simulink model "AR4FullPositionControl"  (R2026a)
settings: Solver=FixedStepAuto  StopTime=inf  FixedStep=3e-5
PreLoadFcn:
  | load('last_pos.mat');
StopFcn:
  | save('last_pos.mat', 'posJ6', 'posJ5', 'posJ4', 'posJ3', 'posJ2', 'posJ1', 'lastX', 'lastY', 'lastZ');
undefined symbols (not defined in the file): targetColor, targetGo, targetX, targetY, targetZ
libraries: arduinolib x31
(part 2 of 3)

== matlab function AR4FullPositionControl/Subsystem/J6/MATLAB Function1 ==
  data: startNext input; clk input; count output; dt input; rst input; displaySpeed output; dir output; pul output; next output; speedRPM input; positionAngle input; currCount input; accelRPMperSec input; limit output; mode input; homed output
function [count, displaySpeed, dir, pul, next, limit, homed] = J6(startNext, clk, dt, rst, speedRPM, positionAngle, currCount, accelRPMperSec, mode)
% J6 - Joint 6 position/speed controller with S-curve acceleration + HOMING
%
% AR4-MK3 robot. Continuous-rotation wrist joint (+/-180 = same physical spot).
% positionAngle is remapped +180 internally. Switch is at count 0.
%
% MODE:
%   0 = POSITION, 1 = INITIALIZE (drive to HOME_TARGET), 2 = HOMING
%
%   >>> maxCount = 20000   GEAR_RATIO = 20000/4000 = 5.0
%   >>> J6 may sit AT the switch (180/-180); limit only flags on TRUE overtravel.

    persistent currentCount lastClkState lastCount spTimer smoothedSpeed ...
               currentRPM distTraveled totalMoveFrozen lastTarget pulseAccum ...
               homedFlag lastMode;

    % -------------------------------------------------------------------------
    % CONSTANTS
    % -------------------------------------------------------------------------
    Ts           = 3e-5;
    PPR          = 1000;
    CPR          = PPR * 4;
    GEAR_RATIO   = 20000 / CPR;
    maxCount     = 20000;
    LIMIT_BUFFER = 5;        % used for homing/fault logic (NOT target clamp)
    TARGET_MARGIN = 0;       % <<< target clamp margin: 0 = allow reaching both ends
    OVERTRAVEL   = 30;       % <<< counts beyond range before a REAL fault trips
    TUNE_C2R     = 0.8;
    C2R          = (GEAR_RATIO * CPR) / 60 * TUNE_C2R;

    speedUpdateInterval = 0.2;
    ALPHA               = 0.3;
    MIN_RPM             = 0.5;
    STOP_COUNTS         = 1;

    HOME_RPM    = 5;    % <<< tune: slow safe homing speed (RPM)
    HOME_TARGET = 0;    % <<< angle commanded in mode=1, for THIS joint (deg)

    % -------------------------------------------------------------------------
    % INITIALISATION (first call only)
    % -------------------------------------------------------------------------
    if isempty(currentCount)
        currentCount    = currCount;
        lastCount       = currCount;
        lastClkState    = clk;
        spTimer         = 0;
        smoothedSpeed   = 0;
        currentRPM      = MIN_RPM;
        distTraveled    = 0;
        totalMoveFrozen = 0;
        lastTarget      = -1;
        pulseAccum      = 0;
        homedFlag       = false;
        lastMode        = 0;
    end

    % Always-assigned outputs
    limit = false;
    homed = homedFlag;
    dir   = 0;
    pul   = 0;
    next  = false;

    % -------------------------------------------------------------------------
    % 1. ENCODER COUNTING  (runs regardless of mode)
    % -------------------------------------------------------------------------
    if clk ~= lastClkState && clk == 1
        if dt ~= clk
            currentCount = currentCount + 1;
        else
            currentCount = currentCount - 1;
        end
    end

    % -------------------------------------------------------------------------
    % RESET S-CURVE STATE ON ANY MODE CHANGE
    % -------------------------------------------------------------------------
    if mode ~= lastMode
        distTraveled    = 0;
        totalMoveFrozen = 0;
        pulseAccum      = 0;
        lastTarget      = -1;
        currentRPM      = MIN_RPM;
        spTimer         = 0;
        smoothedSpeed   = 0;
    end
    lastMode = mode;

    % =========================================================================
    % MODE 2: HOMING  -  drive toward switch, zero count on contact
    % =========================================================================
    if mode == 2

        if rst == 1
            currentCount = 250;
            homedFlag    = true;
        end

        homed = homedFlag;   % switch contact during homing is expected, not a fault

        if homedFlag
            currentCount = 250;
            pul          = 0;
            next         = true;
        elseif startNext
            dir        = 0;   % toward switch = decreasing count
            pulseAccum = pulseAccum + HOME_RPM * C2R * Ts;
            if pulseAccum >= 1.0
                pul        = 1;
                pulseAccum = pulseAccum - 1.0;
            end
        end

        count        = currentCount;
        displaySpeed = HOME_RPM;
        lastClkState = clk;
        return;   % skip position control entirely
    end
    % =========================================================================

    % -------------------------------------------------------------------------
    % 2. SPEED DISPLAY
    % -------------------------------------------------------------------------
    spTimer = spTimer + Ts;
    if spTimer >= speedUpdateInterval
        smoothedSpeed = ALPHA * currentRPM + (1 - ALPHA) * smoothedSpeed;
        spTimer       = 0;
    end

    % -------------------------------------------------------------------------
    % 3. TARGET FROM ANGLE
    % -------------------------------------------------------------------------
    if mode == 1
        cmdAngle = HOME_TARGET;
    else
        cmdAngle = positionAngle;
    end

    cmdAngleRemap = cmdAngle + 180;   % J6 internal remap (+180)
    countsPerDeg  = maxCount / 360;
    targetCount   = round(cmdAngleRemap * countsPerDeg);
    % Allow reaching both ends (0 and maxCount) so 180/-180 are attainable.
    targetCount   = max(TARGET_MARGIN, min(maxCount - TARGET_MARGIN, targetCount));

    % -------------------------------------------------------------------------
    % 4. DIRECTION
    % -------------------------------------------------------------------------
    countError = targetCount - currentCount;
    absError   = abs(countError);

    if countError >= 0
        dir = 1;   % CCW
    else
        dir = 0;   % CW
    end

    % -------------------------------------------------------------------------
    % 5. FREEZE totalMove ON NEW TARGET
    % -------------------------------------------------------------------------
    if targetCount ~= lastTarget
        totalMoveFrozen = absError;
        distTraveled    = 0;
        pulseAccum      = 0;
        lastTarget      = targetCount;
    end

    % -------------------------------------------------------------------------
    % 6. S-CURVE SPEED PROFILE
    % -------------------------------------------------------------------------
    accel = max(accelRPMperSec, 0.1);
    fullRampCounts = 0.5 * (MIN_RPM + speedRPM) * C2R * (speedRPM - MIN_RPM) / accel;

    if totalMoveFrozen > 0 && 2 * fullRampCounts >= totalMoveFrozen
        peakRPM    = sqrt(max(MIN_RPM^2 + totalMoveFrozen * accel / C2R, MIN_RPM^2));
        peakRPM    = max(MIN_RPM, min(speedRPM, peakRPM));
        rampCounts = 0.5 * (MIN_RPM + peakRPM) * C2R * (peakRPM - MIN_RPM) / accel;
        rampCounts = max(1, rampCounts);
    else
        peakRPM    = speedRPM;
        rampCounts = max(1, fullRampCounts);
    end

    if totalMoveFrozen <= 0
        targetRPM = MIN_RPM;
    elseif absError <= rampCounts
        x         = max(0.0, min(1.0, absError / rampCounts));
        targetRPM = MIN_RPM + (peakRPM - MIN_RPM) * 0.5 * (1 - cos(pi * x));
    elseif distTraveled <= rampCounts
        x         = max(0.0, min(1.0, distTraveled / rampCounts));
        targetRPM = MIN_RPM + (peakRPM - MIN_RPM) * 0.5 * (1 - cos(pi * x));
    else
        targetRPM = peakRPM;
    end

    currentRPM = max(MIN_RPM, min(speedRPM, targetRPM));

    % -------------------------------------------------------------------------
    % 7. DDS PULSE ACCUMULATOR
    % -------------------------------------------------------------------------
    if startNext && absError > STOP_COUNTS
        pulseAccum = pulseAccum + currentRPM * C2R * Ts;
        if pulseAccum >= 1.0
            pul          = 1;
            pulseAccum   = pulseAccum - 1.0;
            distTraveled = distTraveled + 1;
        end
        next = false;
    else
        next       = (absError <= STOP_COUNTS);
        pulseAccum = 0;
    end

    % -------------------------------------------------------------------------
    % 8. LIMIT SWITCH SAFETY  -  flag ONLY on true over-travel
    % -------------------------------------------------------------------------
    % Clear homedFlag once we have moved meaningfully away from the switch,
    % so a later genuine over-travel can still be detected.
    if homedFlag && currentCount > LIMIT_BUFFER
        homedFlag = false;
    end

    % TRUE FAULT: only if the joint travels BEYOND the valid count range.
    % Sitting AT the switch (count == 0) or AT the far end (count == maxCount)
    % is allowed and does NOT trip a fault. Only exceeding the range by more
    % than OVERTRAVEL counts is a real fault.
    if currentCount < -OVERTRAVEL
        limit = true;
        pul   = 0;
    end
    if currentCount > (maxCount + OVERTRAVEL)
        limit = true;
        pul   = 0;
    end

    % -------------------------------------------------------------------------
    % 8.5 MODE-0 PULSE SUPPRESSION
    %     In position mode, CoordMove owns all pulse/dir generation.
    %     Force this block's own pul/dir to 0 so it can't leak a second
    %     pulse stream to the driver. Encoder counting + limit safety above
    %     still run normally every tick.
    % -------------------------------------------------------------------------
    if mode == 0
        pul = 0;
    end


    % -------------------------------------------------------------------------
    % 9. OUTPUTS
    % -------------------------------------------------------------------------
    count        = currentCount;
    displaySpeed = smoothedSpeed;
    homed        = homedFlag;
    lastClkState = clk;

end

== matlab function AR4FullPositionControl/Subsystem/MATLAB Function ==
  data: startHoming input; enableIK input; skipHoming input; modeOut output; homed1 input; homed2 input; homed3 input; homed4 input; homed5 input; homed6 input; next1 input; next2 input; next3 input; next4 input; next5 input; next6 input; startNextOut output; stage output; done output
function [modeOut, startNextOut, stage, done] = HomingSequencer( ...
    startHoming, enableIK, skipHoming, ...
    homed1, homed2, homed3, homed4, homed5, homed6, ...
    next1,  next2,  next3,  next4,  next5,  next6)
%HOMINGSEQUENCER  Staged initialization for the AR4 MK3 (paired homing).
%
%   Homes joints in THREE pairs to avoid mechanical cross-coupling
%   (notably J3's zero being disturbed when homed alongside J2):
%       Pair A: J1 & J2
%       Pair B: J3 & J5
%       Pair C: J4 & J6
%
%   Per-pair sequence: HOME to switch (mode 2) -> GOTO home angle (mode 1)
%   -> HOLD at home angle (mode 1) for the rest of calibration.
%
%   mode: 0 = POSITION (IK), 1 = INITIALIZE (drive to HOME_TARGET), 2 = HOMING
%
%   STAGES (phase):
%     0 : IDLE
%     1 : HOME  J1,J2            (wait homed1 & homed2)
%     2 : GOTO  J1,J2 -> home    (wait next1  & next2)
%     3 : HOME  J3,J5            (wait homed3 & homed5)  J1,J2 held
%     4 : GOTO  J3,J5 -> home    (wait next3  & next5)   J1,J2 held
%     5 : HOME  J4,J6            (wait homed4 & homed6)  J1,J2,J3,J5 held
%     6 : GOTO  J4,J6 -> home    (wait next4  & next6)   others held
%     7 : DONE  hold all at home (mode 1) until enableIK -> all mode 0
%
%   INPUTS
%     startHoming - rising edge (0->1) arms the sequence from IDLE
%     enableIK    - when 1 at stage 7, hands control to IK (all mode 0)
%     skipHoming  - when 1, jump straight to stage 7 (DONE) trusting the
%                   already-loaded encoder positions (NO homing performed).
%                   Only safe if the robot's true position is known/loaded.
%     homed1..6   - 'homed' output from each joint block
%     next1..6    - 'next'  output from each joint block
%
%   OUTPUTS (1x6, order J1..J6)
%     modeOut, startNextOut, stage, done

    persistent phase lastStart justEntered lastSkip;

    if isempty(phase)
        phase       = 0;
        lastStart   = 0;
        justEntered = true;
        lastSkip    = 0;
    end

    % -------------------------------------------------------------------------
    % SKIP-HOMING: jump straight to DONE (stage 7) on rising edge of skipHoming
    % Trusts loaded encoder positions; performs no homing motion.
    % -------------------------------------------------------------------------
    if skipHoming == 1 && lastSkip == 0
        phase       = 7;
        justEntered = true;
    end
    lastSkip = skipHoming;

    % -------------------------------------------------------------------------
    % RISING EDGE TRIGGER (normal homing) - only from IDLE
    % -------------------------------------------------------------------------
    if startHoming == 1 && lastStart == 0 && phase == 0
        phase       = 1;
        justEntered = true;
    end
    lastStart = startHoming;

    % -------------------------------------------------------------------------
    % DEFAULTS
    % -------------------------------------------------------------------------
    modeOut      = [0, 0, 0, 0, 0, 0];
    startNextOut = [0, 0, 0, 0, 0, 0];

    % order in arrays: [J1 J2 J3 J4 J5 J6]

    switch phase

        case 0
            % IDLE - waiting for startHoming (or skipHoming) rising edge

        % ================= PAIR A : J1 & J2 =================
        case 1
            % HOME J1, J2
            modeOut      = [2, 2, 0, 0, 0, 0];
            startNextOut = [1, 1, 0, 0, 0, 0];
            if homed1 && homed2
                phase       = 2;
                justEntered = true;
            end

        case 2
            % GOTO J1, J2 -> home angle
            modeOut      = [1, 1, 0, 0, 0, 0];
            startNextOut = [1, 1, 0, 0, 0, 0];
            if justEntered
                justEntered = false;      % skip stale next=true from homing
            elseif next1 && next2
                phase       = 3;
                justEntered = true;
            end

        % ================= PAIR B : J3 & J5 =================
        case 3
            % HOME J3, J5   (J1,J2 held at home angle via mode 1)
            modeOut      = [1, 1, 2, 0, 2, 0];
            startNextOut = [1, 1, 1, 0, 1, 0];
            if homed3 && homed5
                phase       = 4;
                justEntered = true;
            end

        case 4
            % GOTO J3, J5 -> home angle   (J1,J2 still held)
            modeOut      = [1, 1, 1, 0, 1, 0];
            startNextOut = [1, 1, 1, 0, 1, 0];
            if justEntered
                justEntered = false;
            elseif next3 && next5
                phase       = 5;
                justEntered = true;
            end

        % ================= PAIR C : J4 & J6 =================
        case 5
            % HOME J4, J6   (J1,J2,J3,J5 held at home angle)
            modeOut      = [1, 1, 1, 2, 1, 2];
            startNextOut = [1, 1, 1, 1, 1, 1];
            if homed4 && homed6
                phase       = 6;
                justEntered = true;
            end

        case 6
            % GOTO J4, J6 -> home angle   (others still held)
            modeOut      = [1, 1, 1, 1, 1, 1];
            startNextOut = [1, 1, 1, 1, 1, 1];
            if justEntered
                justEntered = false;
            elseif next4 && next6
                phase = 7;
            end

        otherwise
            % STAGE 7: DONE - hold all at home until IK enabled, then hand over
            startNextOut = [1, 1, 1, 1, 1, 1];
            if enableIK
                modeOut = [0, 0, 0, 0, 0, 0];   % IK / positionAngle takes over
            else
                modeOut = [1, 1, 1, 1, 1, 1];   % hold at home position
            end
    end

    stage = phase;
    done  = (phase == 7);

end

== matlab function AR4FullPositionControl/Subsystem/MATLAB Function1 ==
  data: angle1 input; pul1 output; angle2 input; angle3 input; angle4 input; angle5 input; angle6 input; count1 input; count2 input; count3 input; count4 input; count5 input; count6 input; speedRPM input; accelRPMperSec input; pul2 output; pul3 output; pul4 output; pul5 output; pul6 output; dir1 output; dir2 output; dir3 output; dir4 output; dir5 output; dir6 output; enable input; done output
function [pul1, pul2, pul3, pul4, pul5, pul6, ...
          dir1, dir2, dir3, dir4, dir5, dir6, ...
          done] = CoordMove(angle1, angle2, angle3, angle4, angle5, angle6, ...
                            count1, count2, count3, count4, count5, count6, ...
                            speedRPM, accelRPMperSec, enable)
% CoordMove - Coordinated 6-joint motion with single shared S-curve master clock

%
% Replaces per-joint pulse generation in mode=0 (position control).
% J1-J6 blocks still own: encoder counting, homing (mode 2),
% initialize (mode 1), limit safety, and count/homed/limit outputs.
% This block owns: pul and dir for all 6 joints in mode=0 only.
%
% Architecture matches original AR4 firmware (driveMotorsJ):
%   1. Convert target angles -> target counts (per-joint mapping)
%   2. Compute step deltas from current counts
%   3. Find HighStep (limiting joint with most steps)
%   4. Run ONE shared S-curve (accel->cruise->decel) over HighStep ticks
%   5. Each joint fires its pulses proportionally via Bresenham algorithm
%      so all 6 joints arrive together, guaranteed by construction
%
% INPUTS:
%   angle1..6       - target joint angles from IK block (degrees)
%   count1..6       - current encoder counts from J1-J6 blocks
%   speedRPM        - cruise speed for the LIMITING joint (RPM)
%   accelRPMperSec  - acceleration rate (RPM/s)
%   enable          - gate: true = run coordinated move, false = hold
%
% OUTPUTS:
%   pul1..6         - step pulse per joint (0 or 1) -- wire to stepper drivers
%   dir1..6         - direction per joint (0 or 1)  -- wire to stepper drivers
%   done            - true when all joints have reached their targets
%
% WIRING NOTE:
%   In mode=0, wire CoordMove pul/dir outputs to stepper drivers.
%   In mode=1/2, wire J1-J6 pul/dir outputs to stepper drivers instead.
%   Use a Switch block (or Multiport Switch) gated on mode to select.
%   J1-J6 pul/dir outputs in mode=0 can be left disconnected or ignored.

    % -------------------------------------------------------------------------
    % PERSISTENT STATE
    % -------------------------------------------------------------------------
    persistent highStep;           % total master-clock ticks for this move
    persistent masterTick;         % current master-clock tick (0..highStep)
    persistent stepTarget;         % per-joint target step count [1x6]
    persistent dirs;               % per-joint direction [1x6], frozen at move start
    persistent ddaAccum;           % DDA accumulator per joint [1x6] - exact stepping
    persistent targetCountFrozen;  % frozen absolute target count per joint [1x6]
    persistent pulseTarget;        % pulses each joint must fire (countDelta*TUNE) [1x6]
    persistent lastTargetCount;    % frozen target counts from last tick [1x6]
    persistent currentRPM;         % current RPM on the shared S-curve
    persistent C2R_master;         % counts-to-RPM factor for the master (HighStep) joint
    persistent masterAccum;        % DDS accumulator on the master clock
    persistent masterIdx;          % index of the joint that defines highStep
    persistent remSmooth;          % low-pass filtered master remaining pulses
    persistent j5BacklashSign;     % J5 backlash direction, latched per move
    persistent runawayFlag;        % [1x6] joint is moving AWAY from target
    persistent j5LastRawCmd;       % J5 last raw commanded angle (for new-target detect)

    % -------------------------------------------------------------------------
    % PER-JOINT CONSTANTS (from J1-J6 source files)
    % -------------------------------------------------------------------------
    % J1: switch at +170 deg, count increases away from switch
    J1_maxCount    = 37500;  J1_TOTAL_DEG = 340;  J1_SWITCH_DEG =  170;
    J1_LIMIT_BUF   = 50;     J1_TUNE_C2R  = 0.8;
    J1_countsPerDeg = J1_maxCount / J1_TOTAL_DEG;

    % J2: switch at -42 deg, count increases away from switch
    J2_maxCount    = 18300;  J2_TOTAL_DEG = 132;  J2_SWITCH_DEG = -42;
    J2_LIMIT_BUF   = 50;     J2_TUNE_C2R  = 0.8;
    J2_countsPerDeg = J2_maxCount / J2_TOTAL_DEG;

    % J3: switch at +52 deg, count increases away from switch
    J3_maxCount    = 19720;  J3_TOTAL_DEG = 141;  J3_SWITCH_DEG =  52;
    J3_LIMIT_BUF   = 50;     J3_TUNE_C2R  = 0.8;
    J3_countsPerDeg = J3_maxCount / J3_TOTAL_DEG;

    % J4: ZERO_COUNT anchor
    J4_maxCount    = 42860;  J4_TOTAL_DEG = 344;  J4_ZERO_COUNT = 22238;
    J4_LIMIT_BUF   = 50;     J4_TUNE_C2R  = 0.8;
    J4_countsPerDeg = J4_maxCount / J4_TOTAL_DEG;

    % J5: switch at -100 deg, count increases away from switch. Has backlash comp.
    J5_maxCount    = 5800;   J5_TOTAL_DEG = 208.5;  J5_SWITCH_DEG = -100;
    J5_LIMIT_BUF   = 50;     J5_TUNE_C2R  = 1.6;
    J5_J_MIN_DEG   = -100;   J5_J_MAX_DEG = 108.5;
    J5_BACKLASH_DEG = 7.0;   % measured J5 play (must match J5.m)
    J5_countsPerDeg = J5_maxCount / J5_TOTAL_DEG;

    % J6: full rotation, internal +180 remap. TARGET_MARGIN=0 (reaches both ends).
    J6_maxCount    = 20000;
    J6_TARGET_MARGIN = 0;    J6_TUNE_C2R  = 0.8;
    J6_countsPerDeg = J6_maxCount / 360;

    % Per-joint pulse:count ratio (one pulse moves 1/TUNE_C2R encoder counts)
    tuneArr = [J1_TUNE_C2R, J2_TUNE_C2R, J3_TUNE_C2R, ...
               J4_TUNE_C2R, J5_TUNE_C2R, J6_TUNE_C2R];

    % Shared constants
    Ts    = 3e-5;
    CPR   = 1000 * 4;
    MIN_RPM    = 0.5;
    % -------------------------------------------------------------------------
    % PER-JOINT ARRIVAL TOLERANCE
    % Specified in DEGREES (physically meaningful) and converted to counts,
    % because counts/deg varies 5x across joints (J5 ~28, J3 ~140).
    %
    % +/-3 counts asks for repeatability the mechanism does not have: for J1
    % that is 0.027 deg. After its last pulse a joint settles back a few counts
    % from backlash/compliance, and since one pulse moves ~1.25 counts it lands
    % on a discrete grid. Usually inside the band, occasionally not -- which is
    % why every joint fails sometimes and J4 (most lash, smallest moves) fails
    % most.
    %
    % Tolerances are chosen by ROLE, not uniformly:
    %   J1,J2,J3 positioning -> tight, these set TCP position directly
    %   J5       wrist pitch -> moderate, sets gripper tilt
    %   J4,J6    rolls       -> loose, only affect gripper YAW, which is
    %                          immaterial for a straight-down gripper
    % -------------------------------------------------------------------------
    TOL_DEG_J1 = 0.15;   % ~17 counts  (~1.0 mm TCP at 400 mm reach)
    TOL_DEG_J2 = 0.15;   % ~21 counts
    TOL_DEG_J3 = 0.15;   % ~21 counts
    TOL_DEG_J4 = 1.00;   % ~125 counts (roll: yaw only)
    TOL_DEG_J5 = 0.30;   % ~8 counts
    TOL_DEG_J6 = 1.00;   % ~56 counts  (roll: yaw only)

    MIN_STOP_COUNTS = 3; % floor: never tighter than ~2x one pulse's movement

    % RUNAWAY GUARD: if a joint's error ever exceeds the distance it was asked
    % to travel by this margin, it is moving AWAY from target -- its direction
    % sense is wrong. Stop pulsing that joint rather than driving it into a
    % hard limit. 'done' will not fire, which is the correct, visible failure.
    RUNAWAY_MARGIN = 400;   % counts (~3.2 deg on J4, ~3.6 deg on J1)

    % ACC/DCC ramp fraction of total move (matching original firmware defaults)
    ACC_FRAC = 0.25;   % 25% of move for accel ramp
    DCC_FRAC = 0.25;   % 25% of move for decel ramp

    % -------------------------------------------------------------------------
    % INITIALISATION (first call only)
    % -------------------------------------------------------------------------
    if isempty(highStep)
        highStep        = 0;
        masterTick      = 0;
        stepTarget      = zeros(1,6);
        dirs            = zeros(1,6);
        ddaAccum        = zeros(1,6);
        targetCountFrozen = zeros(1,6);
        pulseTarget       = zeros(1,6);
        lastTargetCount = zeros(1,6);
        currentRPM      = MIN_RPM;
        C2R_master      = 1;
        masterAccum     = 0;
        masterIdx       = 1;
        remSmooth       = 0;
        j5BacklashSign  = 0;
        j5LastRawCmd    = -999;   % force first J5 target to register as new
        runawayFlag     = false(1,6);
    end

    % Default outputs every tick (Simulink requires all outputs assigned)
    pul1 = 0; pul2 = 0; pul3 = 0; pul4 = 0; pul5 = 0; pul6 = 0;
    dir1 = dirs(1); dir2 = dirs(2); dir3 = dirs(3);
    dir4 = dirs(4); dir5 = dirs(5); dir6 = dirs(6);
    done = 0;

    if ~enable
        done = 0;
        return;
    end

    % -------------------------------------------------------------------------
    % 1. ANGLE -> TARGET COUNT (matching each J-file's own mapping exactly)
    % -------------------------------------------------------------------------
    % J1: single-limit, switch-anchored at +170
    tc1 = round(abs(J1_SWITCH_DEG - angle1) * J1_countsPerDeg);
    tc1 = max(J1_LIMIT_BUF, min(J1_maxCount - J1_LIMIT_BUF, tc1));

    % J2: single-limit, switch-anchored at -42 (moving away increases count)
    tc2 = round(abs(J2_SWITCH_DEG - angle2) * J2_countsPerDeg);
    tc2 = max(J2_LIMIT_BUF, min(J2_maxCount - J2_LIMIT_BUF, tc2));

    % J3: single-limit, switch-anchored at +52
    tc3 = round(abs(J3_SWITCH_DEG - angle3) * J3_countsPerDeg);
    tc3 = max(J3_LIMIT_BUF, min(J3_maxCount - J3_LIMIT_BUF, tc3));

    % J4: ZERO_COUNT anchor
    tc4 = round(J4_ZERO_COUNT + angle4 * J4_countsPerDeg);
    tc4 = max(J4_LIMIT_BUF, min(J4_maxCount - J4_LIMIT_BUF, tc4));

    % J5: single-limit, switch-anchored at -100, WITH backlash compensation.
    % Must replicate J5.m exactly: latch backlash direction on a new target
    % based on travel direction from current physical position, then HOLD it.
    j5HalfBacklash = J5_BACKLASH_DEG / 2;
    j5RawTarget    = angle5;                 % uncompensated commanded angle

    if abs(j5RawTarget - j5LastRawCmd) > 0.5   % a NEW target was commanded
        j5CurrentAngle = J5_SWITCH_DEG + (count5 / J5_countsPerDeg);
        if j5RawTarget > j5CurrentAngle
            j5BacklashSign = 1;
        elseif j5RawTarget < j5CurrentAngle
            j5BacklashSign = -1;
        else
            j5BacklashSign = 0;
        end
        j5LastRawCmd = j5RawTarget;
    end

    j5CmdAngle = j5RawTarget + j5BacklashSign * j5HalfBacklash;
    if j5CmdAngle < J5_J_MIN_DEG, j5CmdAngle = J5_J_MIN_DEG; end
    if j5CmdAngle > J5_J_MAX_DEG, j5CmdAngle = J5_J_MAX_DEG; end
    tc5 = round(abs(J5_SWITCH_DEG - j5CmdAngle) * J5_countsPerDeg);
    tc5 = max(J5_LIMIT_BUF, min(J5_maxCount - J5_LIMIT_BUF, tc5));

    % J6: full rotation, internal +180 remap
    tc6 = round((angle6 + 180) * J6_countsPerDeg);
    tc6 = max(J6_TARGET_MARGIN, min(J6_maxCount - J6_TARGET_MARGIN, tc6));

    newTargetCounts = [tc1, tc2, tc3, tc4, tc5, tc6];
    currentCounts   = [count1, count2, count3, count4, count5, count6];

    % -------------------------------------------------------------------------
    % 2. NEW MOVE DETECTION
    %    If target counts changed from last tick, freeze everything and
    %    set up a fresh move. Matching the J-file "lastTarget" pattern.
    % -------------------------------------------------------------------------
    targetChanged = any(newTargetCounts ~= lastTargetCount);

    if targetChanged
        % Per-joint count deltas
        deltas     = newTargetCounts - currentCounts;
        stepTarget = abs(deltas);          % counts each joint must travel

        % ---------------------------------------------------------------
        % PULSE-BASED DDA SIZING (fixes J5 lag / arrives-late bug)
        % Each pulse moves the encoder 1/TUNE_C2R counts, so the number of
        % PULSES a joint needs is countDelta * TUNE_C2R. J5 (TUNE=1.6) needs
        % MORE pulses per count than the others (TUNE=0.8); if the DDA is
        % sized in raw counts, J5 is starved of pulses and finishes late.
        % Distribute the DDA by PULSES NEEDED so all joints finish together.
        % ---------------------------------------------------------------
        pulseTarget = zeros(1,6);
        for i = 1:6
            pulseTarget(i) = round(stepTarget(i) * tuneArr(i));
        end

        % highStep = max PULSES across joints (limiting joint sets duration).
        % DDA increment pulseTarget(i) <= highStep guarantees <=1 pulse/tick.
        highStep = double(max(pulseTarget(:)));

        % C2R per joint (pulse-rate factor, includes per-joint TUNE_C2R)
        c2r_all = zeros(1,6);
        c2r_all(1) = ((J1_maxCount/J1_TOTAL_DEG*360)/CPR * CPR)/60 * J1_TUNE_C2R;
        c2r_all(2) = ((J2_maxCount/J2_TOTAL_DEG*360)/CPR * CPR)/60 * J2_TUNE_C2R;
        c2r_all(3) = ((J3_maxCount/J3_TOTAL_DEG*360)/CPR * CPR)/60 * J3_TUNE_C2R;
        c2r_all(4) = ((J4_maxCount/J4_TOTAL_DEG*360)/CPR * CPR)/60 * J4_TUNE_C2R;
        c2r_all(5) = ((J5_maxCount/J5_TOTAL_DEG*360)/CPR * CPR)/60 * J5_TUNE_C2R;
        c2r_all(6) = ((J6_maxCount/360      *360)/CPR * CPR)/60 * J6_TUNE_C2R;

        % Master clock rate from the joint with the most PULSES
        masterJoint = 1;
        for mj = 1:6
            if pulseTarget(mj) >= pulseTarget(masterJoint)
                masterJoint = mj;
            end
        end
        C2R_master = c2r_all(masterJoint);
        masterIdx  = masterJoint;              % joint that defines the timebase
        remSmooth  = double(pulseTarget(masterJoint));   % seed = full move

        % Reset master clock and per-joint DDA counters
        masterTick = 0;
        ddaAccum   = zeros(1,6);
        currentRPM = MIN_RPM;

        runawayFlag = false(1,6);      % fresh move, nobody is running away yet

        % Freeze absolute target counts for encoder-based stop
        targetCountFrozen = newTargetCounts;

        lastTargetCount = newTargetCounts;
    end

    % -------------------------------------------------------------------------
    % 3. PER-TICK DIRECTION SERVO + ENCODER-BASED STOP
    %    Direction is recomputed EVERY tick from live encoder error (like the
    %    J-blocks), so a joint that overshoots reverses and settles instead of
    %    running away. "Reached" is within STOP_COUNTS. The DDA (below) still
    %    governs coordinated TIMING; this only governs direction + stop.
    %
    %    countError(i) = targetCountFrozen(i) - liveCount(i)
    %    Per-joint dir convention (from each J-file, NOT uniform):
    %      J1: err>=0 -> dir=1 | J2: err>=0 -> dir=1 | J3: err>=0 -> dir=0
    %      J4: err>=0 -> dir=1 | J5: err>=0 -> dir=1 | J6: err>=0 -> dir=1
    % -------------------------------------------------------------------------
    liveCounts   = [count1, count2, count3, count4, count5, count6];
    jointReached = false(1,6);
    countErr     = zeros(1,6);
    % Per-joint arrival tolerance: degrees -> counts, floored
    stopBand = zeros(1,6);
    stopBand(1) = max(MIN_STOP_COUNTS, round(TOL_DEG_J1 * J1_countsPerDeg));
    stopBand(2) = max(MIN_STOP_COUNTS, round(TOL_DEG_J2 * J2_countsPerDeg));
    stopBand(3) = max(MIN_STOP_COUNTS, round(TOL_DEG_J3 * J3_countsPerDeg));
    stopBand(4) = max(MIN_STOP_COUNTS, round(TOL_DEG_J4 * J4_countsPerDeg));
    stopBand(5) = max(MIN_STOP_COUNTS, round(TOL_DEG_J5 * J5_countsPerDeg));
    stopBand(6) = max(MIN_STOP_COUNTS, round(TOL_DEG_J6 * J6_countsPerDeg));

    for i = 1:6
        countErr(i) = targetCountFrozen(i) - liveCounts(i);
        if abs(countErr(i)) <= stopBand(i)
            jointReached(i) = true;
        end
    end

    % Runaway detection: error larger than the commanded travel + margin means
    % this joint is being driven the wrong way.
    for i = 1:6
        if abs(countErr(i)) > (stepTarget(i) + RUNAWAY_MARGIN)
            runawayFlag(i) = true;
        end
    end

    % Recompute direction each tick (servo). Convention per joint.
    if countErr(1) >= 0, dirs(1) = 1; else, dirs(1) = 0; end   % J1
    if countErr(2) >= 0, dirs(2) = 1; else, dirs(2) = 0; end   % J2
    if countErr(3) >= 0, dirs(3) = 0; else, dirs(3) = 1; end   % J3
    if countErr(4) >= 0, dirs(4) = 1; else, dirs(4) = 0; end   % J4
    if countErr(5) >= 0, dirs(5) = 1; else, dirs(5) = 0; end   % J5
    if countErr(6) >= 0, dirs(6) = 1; else, dirs(6) = 0; end   % J6

    if highStep <= 0 || all(jointReached)
        done = 1;
        dir1 = dirs(1); dir2 = dirs(2); dir3 = dirs(3);
        dir4 = dirs(4); dir5 = dirs(5); dir6 = dirs(6);
        return;
    end

    % -------------------------------------------------------------------------
    % 4. SHARED S-CURVE: compute currentRPM for this master tick
    %    One accel->cruise->decel profile driven by masterTick vs highStep.
    %    Uses same cosine-blend S-curve shape as J1-J6 blocks for consistency.
    % -------------------------------------------------------------------------
    ACCStep = highStep * ACC_FRAC;
    DCCStep = highStep * DCC_FRAC;

    % fullRampCounts: how many master ticks a full accel ramp takes at speedRPM
    accel = max(accelRPMperSec, 0.1);
    fullRampCounts = 0.5 * (MIN_RPM + speedRPM) * C2R_master * (speedRPM - MIN_RPM) / accel;

    % If move is short, reduce peakRPM so ramps fit
    if highStep > 0 && 2 * fullRampCounts >= highStep
        peakRPM = sqrt(max(MIN_RPM^2 + highStep * accel / C2R_master, MIN_RPM^2));
        peakRPM = max(MIN_RPM, min(speedRPM, peakRPM));
        rampCounts = 0.5*(MIN_RPM+peakRPM)*C2R_master*(peakRPM-MIN_RPM)/accel;
        rampCounts = max(1, rampCounts);
    else
        peakRPM    = speedRPM;
        rampCounts = max(1, fullRampCounts);
    end

    % ---------------------------------------------------------------------
    % SELF-CORRECTING DECEL (mirrors the J-file method)
    %
    % Decel is driven by the MASTER joint's LIVE remaining error, converted to
    % pulses, instead of (highStep - masterTick). This makes the profile
    % closed-loop like the J-blocks: if the joint lags, decel waits; if it
    % arrives early, decel is already finished. masterTick can no longer run
    % past highStep and pin the clock at MIN_RPM.
    %
    % Only the MASTER joint's error is used -- deliberately NOT max() across
    % all six. A max() switches which joint it tracks mid-move, which makes the
    % signal jump and destroys smoothness. One joint = one monotonic signal.
    %
    % Encoder counts are integers, so the raw signal is quantised; it is
    % low-pass filtered (same idea as ALPHA on displaySpeed in the J-files)
    % so the ramp glides instead of stepping.
    % ---------------------------------------------------------------------
    REM_ALPHA = 0.02;   % smoothing on the measured error (smaller = smoother)

    remRaw    = abs(countErr(masterIdx)) * tuneArr(masterIdx);   % pulses to go
    remSmooth = remSmooth + REM_ALPHA * (remRaw - remSmooth);

    % Decel checked FIRST (as the J-files do): arrival always wins over ramp-up.
    if remSmooth <= rampCounts
        x = max(0.0, min(1.0, remSmooth / rampCounts));
        targetRPM = MIN_RPM + (peakRPM - MIN_RPM) * 0.5 * (1 - cos(pi * x));
    elseif masterTick <= rampCounts
        x = max(0.0, min(1.0, masterTick / rampCounts));
        targetRPM = MIN_RPM + (peakRPM - MIN_RPM) * 0.5 * (1 - cos(pi * x));
    else
        targetRPM = peakRPM;
    end
    currentRPM = max(MIN_RPM, min(speedRPM, targetRPM));

    % -------------------------------------------------------------------------
    % 5. MASTER TICK: should we fire a pulse this Simulink timestep?
    %    DDS accumulator on the MASTER clock only.
    %    Each Simulink tick, accumulate currentRPM * C2R_master * Ts.
    %    When accumulator >= 1.0, fire one master tick and run Bresenham.
    % -------------------------------------------------------------------------
    if targetChanged
        masterAccum = 0;
    end

    masterAccum = masterAccum + currentRPM * C2R_master * Ts;

    if masterAccum < 1.0
        % No master tick this Simulink timestep — hold outputs
        dir1 = dirs(1); dir2 = dirs(2); dir3 = dirs(3);
        dir4 = dirs(4); dir5 = dirs(5); dir6 = dirs(6);
        return;
    end
    masterAccum = masterAccum - 1.0;
    masterTick  = masterTick + 1;

    % -------------------------------------------------------------------------
    % 6. DDA PROPORTIONAL STEPPING with ENCODER-BASED STOP
    %    The DDA governs proportional TIMING (keeps joints coordinated), but a
    %    joint stops firing once its LIVE encoder count reaches target -- NOT
    %    when a pulse tally is met. This self-corrects for pulse:count ratio
    %    (TUNE_C2R etc.), exactly like the individual J-blocks do.
    % -------------------------------------------------------------------------
    pulses = zeros(1,6);

    for i = 1:6
        if jointReached(i)
            continue;                      % encoder reached target -> stop
        end
        if runawayFlag(i)
            continue;                      % wrong direction -> refuse to drive
        end

        % A joint that is NOT yet reached must always be able to step. If its
        % frozen pulseTarget rounded to 0 (its delta was ~0 when the move was
        % set up) the old code skipped it forever, so it could never correct
        % drift and 'done' could never fire. Give it the full rate instead.
        inc = pulseTarget(i);
        if inc <= 0
            inc = highStep;
        end

        ddaAccum(i) = ddaAccum(i) + inc;
        if ddaAccum(i) >= highStep
            ddaAccum(i) = ddaAccum(i) - highStep;
            pulses(i)   = 1;               % fire a step this tick
        end
    end

    % -------------------------------------------------------------------------
    % 7. ASSIGN OUTPUTS
    % -------------------------------------------------------------------------
    pul1 = pulses(1); pul2 = pulses(2); pul3 = pulses(3);
    pul4 = pulses(4); pul5 = pulses(5); pul6 = pulses(6);
    dir1 = dirs(1);   dir2 = dirs(2);   dir3 = dirs(3);
    dir4 = dirs(4);   dir5 = dirs(5);   dir6 = dirs(6);

    done = double(all(jointReached));

end

== matlab function AR4FullPositionControl/MATLAB Function2 ==
  data: targetX input; cmdX output; targetY input; targetZ input; targetColor input; newTarget input; moveComplete input; cmdY output; cmdZ output; gripperClose output; done output; state output
function [cmdX, cmdY, cmdZ, gripperClose, done, state] = pickPlaceFSM(...
        targetX, targetY, targetZ, targetColor, newTarget, moveComplete)
%#codegen
% Pick-and-place FSM. Outputs a Cartesian target for the IK block and
% advances one state only after the commanded move has GENUINELY completed.
%
% MOVE DETECTION -- two-phase handshake (see notes in prior version):
%   phase 0 = wait for move to START (signal LOW, or START_TIMEOUT for
%             near-zero moves), phase 1 = wait to SETTLE (high for
%             STABLE_STEPS). MOVE_TIMEOUT is a hard safety cap.
%   moveComplete should be CoordMove's encoder-based done, NOT pathStep done.
%
% COLOR SORTING: targetColor is latched alongside the target coordinates at
% pickup time (objColor), so a mid-cycle change to the pushed parameter can
% never re-route a block already in the gripper. S_PLACE_A / S_PLACE_B are
% separate states so each drop-off can be tuned independently later.

    Ts = 0.03;   % must match this block's actual sample time (s)

    % Setpoints [x y z] mm, robot base frame
    INTERMEDIATE = [-50, 350, 220];    % fill with real values
    PLACE_A      = [-100, 250, 220];   % drop-off for color 1  
    PLACE_B      = [0, 250, 220];      % drop-off for color 2  
    HOME         = [-50, 250, 220];
    CAM          = [-50, 250, 220];
    HOVER_OFF    = 40;

    GRIP_CLOSE_DWELL = round(0.8 / Ts);
    GRIP_OPEN_DWELL  = round(0.8 / Ts);

    % Move handshake timing (all in samples)
    START_TIMEOUT = round(0.50 / Ts);   % if signal never drops, assume started
    STABLE_STEPS  = round(0.20 / Ts);   % continuous-high to count as settled
    MOVE_TIMEOUT  = round(6.0  / Ts);   % hard safety cap per move-state

    S_WAIT=1; S_HOVER=2; S_PICK=3; S_CLOSE=4; S_LIFT=5;
    S_INTER=6; S_PLACE_A=7; S_OPEN=8; S_HOME=9; S_PLACE_B=10;

    persistent st cmd objX objY objZ objColor dwell stableCnt phase
    if isempty(st)
        st = S_WAIT; cmd = CAM;
        objX = 0; objY = 0; objZ = 150; objColor = 1;
        dwell = 0; stableCnt = 0;
        phase = 0;                 % 0 = waiting for move to START, 1 = waiting to SETTLE
    end

    % Settle debounce
    if moveComplete
        stableCnt = stableCnt + 1;
    else
        stableCnt = 0;
    end

    dwell = dwell + 1;             % samples since this state (move) was entered

    if phase == 0
        if (~moveComplete) || (dwell >= START_TIMEOUT)
            phase = 1;             % move has started (or assumed started)
            stableCnt = 0;         % reset settle debounce for the settle phase
        end
    end

    moveDoneStable = false;
    if phase == 1 && stableCnt >= STABLE_STEPS
        moveDoneStable = true;
    end
    if dwell >= MOVE_TIMEOUT
        moveDoneStable = true;     % safety fallback -- never hang
    end

    gripperClose = 0;
    done = 0;

    switch st
        case S_WAIT                         % at camera pose, gripper open
            cmd = CAM; gripperClose = 0;
            if moveDoneStable
                done = 1;
                if newTarget
                    objX = targetX; objY = targetY; objZ = targetZ;
                    objColor = targetColor;         % latch color with the target
                    cmd = [objX, objY, objZ + HOVER_OFF];
                    st = S_HOVER; dwell = 0; stableCnt = 0; phase = 0; done = 0;
                end
            end

        case S_HOVER                        % above object
            gripperClose = 0;
            if moveDoneStable
                cmd = [objX, objY, objZ];   % descend onto object
                st = S_PICK; dwell = 0; stableCnt = 0; phase = 0;
            end

        case S_PICK                         % down onto object
            gripperClose = 0;
            if moveDoneStable
                st = S_CLOSE; dwell = 0; stableCnt = 0; phase = 0;
            end

        case S_CLOSE                        % grip, hold, wait (no move)
            gripperClose = 1;
            if dwell >= GRIP_CLOSE_DWELL
                cmd = [objX, objY, objZ + HOVER_OFF];   % lift straight up
                st = S_LIFT; dwell = 0; stableCnt = 0; phase = 0;
            end

        case S_LIFT
            gripperClose = 1;
            if moveDoneStable
                cmd = INTERMEDIATE;
                st = S_INTER; dwell = 0; stableCnt = 0; phase = 0;
            end

        case S_INTER                        % route by latched color
            gripperClose = 1;
            if moveDoneStable
                if objColor == 2
                    cmd = PLACE_B;
                    st = S_PLACE_B;
                else
                    cmd = PLACE_A;          
                    st = S_PLACE_A;
                end
                dwell = 0; stableCnt = 0; phase = 0;
            end

        case S_PLACE_A                      % drop-off for color 1
            gripperClose = 1;
            if moveDoneStable
                st = S_OPEN; dwell = 0; stableCnt = 0; phase = 0;
            end

        case S_PLACE_B                      % drop-off for color 2
            gripperClose = 1;
            if moveDoneStable
                st = S_OPEN; dwell = 0; stableCnt = 0; phase = 0;
            end

        case S_OPEN                         % release, wait (no move)
            gripperClose = 0;
            if dwell >= GRIP_OPEN_DWELL
                cmd = HOME;
                st = S_HOME; dwell = 0; stableCnt = 0; phase = 0;
            end

        case S_HOME
            gripperClose = 0;
            if moveDoneStable
                st = S_WAIT; dwell = 0; stableCnt = 0; phase = 0;
            end

        otherwise
            st = S_WAIT; cmd = CAM;
    end

    cmdX = cmd(1); cmdY = cmd(2); cmdZ = cmd(3);
    state = st;
end
